simulink model "Control_feedback"  (R2024b)
settings: Solver=VariableStepAuto  StartTime=0.0  StopTime=10.0  RelTol=1e-3
values from neighbouring files (symbols this model uses):
  Kb = 1.00    (= 1)    [controller_workspace.m]
  Kp = 4.47    [controller_workspace.m]
  y = 1    [controller_workspace.m]
undefined symbols (not defined in the file or in its folder): DiscIntNeverNeededParam, Discrete, r, Time
libraries: ctrlSharedLib x1
settings Model: Creator=vivek  LastModifiedBy=vivek

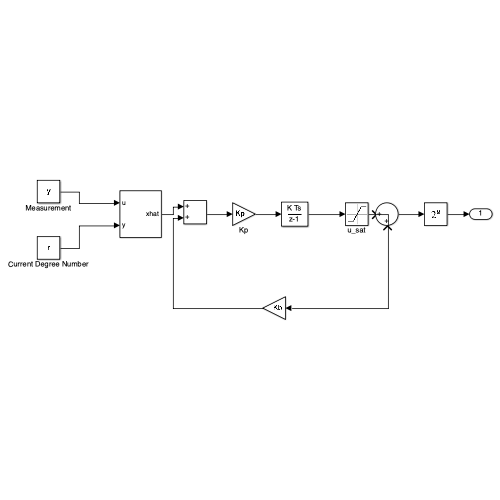
[thumbnail: Simulink's stored preview of the top-level diagram]
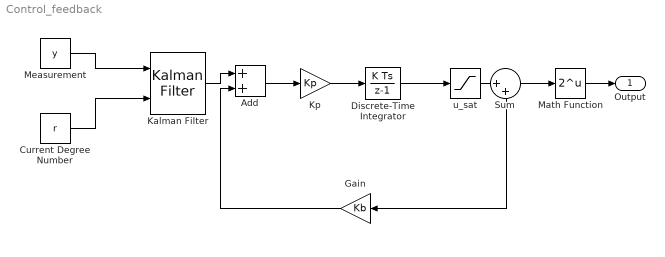
== system Control_feedback ==
  Add : Sum
  Current Degree Number : Constant  Value=r
  Discrete-Time Integrator : DiscreteIntegrator  gainval=0.167  SampleTime=-1  ICPrevOutput=DiscIntNeverNeededParam  ICPrevScaledInput=DiscIntNeverNeededParam
  Gain : Gain  Gain=Kb
  Kalman Filter : ctrlSharedLib/Kalman Filter  TimeDomain=Discrete-Time  UseCurrentEstimator=on  ModelSource=LTI State-Space Variable  ModelSourceVariable=ss(0.95,1,1,0,1)  A=0.95  B=1  C=1  D=0  NumberOfStates=1  NumberOfInputs=1  NumberOfOutputs=1  InitialEstimateSource=Dialog  X0=0  P0=10  UseK=off  UseGH=off  NumberOfProcessNoiseInputs=1  G=1  TimeInvariantG=on  H=0  TimeInvariantH=on  Q=0.05  TimeInvariantQ=on  R=1  TimeInvariantR=on  N=0  TimeInvariantN=on  AddInputPort=on  AddEnablePort=off  OutputEstimatedY=off  OutputP=off  Ts=-1
  Kp : Gain  Gain=Kp
  Math Function : Math  Operator=2^u
  Measurement : Constant  Value=y
  Sum : Sum  Inputs=|++
  u_sat : Saturate  UpperLimit=270  LowerLimit=0
  Output : Outport
  wires:
  Current Degree Number/1 -> Kalman Filter/2
  Measurement/1 -> Kalman Filter/1
  Kalman Filter/1 -> Add/1
  Add/1 -> Kp/1
  Kp/1 -> Discrete-Time Integrator/1
  Discrete-Time Integrator/1 -> u_sat/1
  Gain/1 -> Add/2
  u_sat/1 -> Gain/1
  Sum/1 -> Math Function/1
  Math Function/1 -> Output/1
